simulink model "mcb_microchip_pmsm_foc_sensorless_SAME54"  (R2023b)
settings: Solver=FixedStepDiscrete  StartTime=0.0  StopTime=5  FixedStep=Ts  RelTol=1e-3  EnableMultiTasking=on
InitFcn:
  | mcb_microchip_pmsm_foc_sensorless_SAME54_data
values from neighbouring files (symbols this model uses):
  PI_params = mcb.internal.SetControllerParameters(pmsm,inverter,PU_System,T_pwm,2*Ts,Ts_speed)    [mcb_microchip_pmsm_foc_sensorless_SAME54_data.m]
  PU_System = mcb_SetPUSystem(pmsm,inverter)    [mcb_microchip_pmsm_foc_sensorless_SAME54_data.m]
  PWM_frequency = 12e3    (= 12000)    [mcb_microchip_pmsm_foc_sensorless_SAME54_data.m]
  Ts = T_pwm    (= 8.33333333333e-05)    [mcb_microchip_pmsm_foc_sensorless_SAME54_data.m]
  Ts_motor = T_pwm    (= 8.33333333333e-05)    [mcb_microchip_pmsm_foc_sensorless_SAME54_data.m]
  Ts_simulink = T_pwm    (= 8.33333333333e-05)    [mcb_microchip_pmsm_foc_sensorless_SAME54_data.m]
  Ts_speed = 10*Ts    (= 0.000833333333333)    [mcb_microchip_pmsm_foc_sensorless_SAME54_data.m]
  Vd_Ref_openLoop_PU = 0.15    [mcb_microchip_pmsm_foc_sensorless_SAME54_data.m]
undefined symbols (not defined in the file or in its folder): AIN0, AIN6, DiscIntNeverNeededParam, inverter, PA02, PA03, PA06, PA08, PA09, PA10, PA11, PA12, PA13, PA16, PA17, PA18, pad0, pad1, pad2, pad3, PB08, Pin, pmsm, SAME54P20A, Timer, TQFP128, VREFA, wo0, wo1, wo2, wo4, wo5, wo6
libraries: simulink x15, MCHP_Blockset x12, mcbcontrolslib x10, slpidlib x3, mcbpositiondecoderlib x2, mcbplantlib x1, autolibpmsmexterior x1
(part 3 of 4)

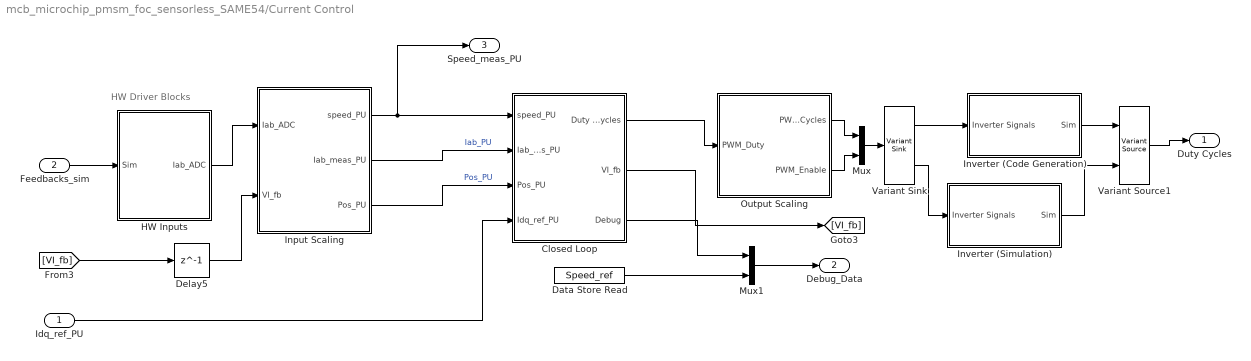
== system mcb_microchip_pmsm_foc_sensorless_SAME54/Current Control ==
  note: HW Driver Blocks
  Idq_ref_PU : Inport
  Feedbacks_sim : Inport  Port=2
  Closed Loop : Subsystem
  Data Store Read : DataStoreRead  DataStoreName=Speed_ref  DataStoreElements=Speed_ref  IndexOptions=Index vector (dialog)  Indices=1  OutputSizes=1
  Delay5 : Delay  DelayLength=1  SampleTime=Ts
  HW Inputs : Subsystem  Variant=on  VariantControlMode=sim codegen switching
  Input Scaling : Subsystem
  Inverter (Code Generation) : Subsystem
  Inverter (Simulation) : Subsystem
  Mux : Mux  Inputs=2
  Mux1 : Mux  Inputs=2
  Output Scaling : Subsystem
  Variant Sink : VariantSink  VariantControlMode=sim codegen switching
  Variant Source1 : VariantSource  VariantControlMode=sim codegen switching
  Duty Cycles : Outport  InitialOutput=0  VectorParamsAs1DForOutWhenUnconnected=off
  Debug_Data : Outport  Port=2
  Speed_meas_PU : Outport  Port=3  InitialOutput=0  VectorParamsAs1DForOutWhenUnconnected=off
  wires:
  Output Scaling/2(PWM_Enable) -> Mux/2
  Feedbacks_sim/1 -> HW Inputs/1(Sim)
  Input Scaling/2(Iab_meas_PU) -> Closed Loop/2(Iab_meas_PU)  "Iab_PU"
  Input Scaling/3(Pos_PU) -> Closed Loop/3(Pos_PU)  "Pos_PU"
  Variant Source1/1 -> Duty Cycles/1
  Output Scaling/1(PWM_Duty_Cycles) -> Mux/1
  Variant Sink/2 -> Inverter (Simulation)/1(Inverter Signals)
  Inverter (Code Generation)/1(Sim) -> Variant Source1/1
  Inverter (Simulation)/1(Sim) -> Variant Source1/2
  Variant Sink/1 -> Inverter (Code Generation)/1(Inverter Signals)
  Mux/1 -> Variant Sink/1
  HW Inputs/1(Iab_ADC) -> Input Scaling/1(Iab_ADC)
  [VI_fb] -> Delay5/1
  Delay5/1 -> Input Scaling/2(VI_fb)
  Mux1/1 -> Debug_Data/1
  Data Store Read/1 -> Mux1/2
  Input Scaling/1(speed_PU) -> Closed Loop/1(speed_PU), Speed_meas_PU/1
  Idq_ref_PU/1 -> Closed Loop/4(Idq_ref_PU)
  Closed Loop/1(Duty Cycles) -> Output Scaling/1(PWM_Duty)
  Closed Loop/2(VI_fb) -> [VI_fb]
  Closed Loop/3(Debug) -> Mux1/1

== system mcb_microchip_pmsm_foc_sensorless_SAME54/Heartbeat LED ==
  note: Heartbeat LED 1HZ
  Code generation : Subsystem
  RED_LED : Constant  OutDataTypeStr=uint16  SampleTime=0.1
  Simulation : Subsystem
  Variant Sink : VariantSink
  wires:
  RED_LED/1 -> Variant Sink/1
  Variant Sink/1 -> Code generation/1(In1)
  Variant Sink/2 -> Simulation/1(In1)

== system mcb_microchip_pmsm_foc_sensorless_SAME54/Inverter and Motor - Plant Model ==
  Duty_Cycles : Inport
  Plant Model : Subsystem  Variant=on  VariantControlMode=sim codegen switching  VariantControl=Variant1  PropagateVariantConditions=on
  Feedbacks_sim : Outport  VectorParamsAs1DForOutWhenUnconnected=off
  wires:
  Duty_Cycles/1 -> Plant Model/1(Duty_Cycles)
  Plant Model/1(Feedbacks_sim) -> Feedbacks_sim/1

== system mcb_microchip_pmsm_foc_sensorless_SAME54/Serial Receive ==
  CodeGen : Subsystem
  Data Store Write : DataStoreWrite  DataStoreName=Enable  IndexOptions=Index vector (dialog)  Indices=1  OutputSizes=1
  Sim : Subsystem
  Variant Source : VariantSource  VariantControlMode=sim codegen switching
  Variant Source1 : VariantSource  VariantControlMode=sim codegen switching
  SpeedRef : Outport
  wires:
  Variant Source/1 -> SpeedRef/1
  Variant Source1/1 -> Data Store Write/1
  Sim/1(SpeedRef) -> Variant Source/2
  Sim/2(Enable) -> Variant Source1/2
  CodeGen/1(SpeedRef) -> Variant Source/1
  CodeGen/2(Enable) -> Variant Source1/1

== system mcb_microchip_pmsm_foc_sensorless_SAME54/Speed Control ==
  SpeedRef : Inport
  Speed_Meas_PU : Inport  Port=2
  Data Store Write3 : DataStoreWrite  DataStoreName=Speed_ref  IndexOptions=Index vector (dialog)  Indices=1  OutputSizes=1
  Id_Ref : Constant  Value=0  OutDataTypeStr=dataType
  Mux : Mux  Inputs=2
  PI_Controller_Speed : Subsystem
  Speed_Ref_Selector : Subsystem
  IdqRef_PU : Outport  VectorParamsAs1DForOutWhenUnconnected=off
  wires:
  PI_Controller_Speed/1(Iq_ref) -> Mux/2
  Speed_Meas_PU/1 -> PI_Controller_Speed/2(N_fb)  "Speed_fb"
  Id_Ref/1 -> Mux/1
  Mux/1 -> IdqRef_PU/1
  Speed_Ref_Selector/1(Speed_Ref1) -> PI_Controller_Speed/1(N_ref)  "Speed_ref"
  SpeedRef/1 -> Data Store Write3/1, Speed_Ref_Selector/1(Speed_Ref)

== system mcb_microchip_pmsm_foc_sensorless_SAME54/Subsystem2 ==
  note: Fast Serial Data Monitoring (32-bit)
  Data_Log : Inport
  Counter Limited : simulink/Sources/Counter Limited  uplimit=59  tsamp=Ts_SerialCom
  Data : Subsystem  TreatAsAtomicUnit=on
  End : Subsystem  TreatAsAtomicUnit=on
  If : If  IfExpression=u1 == 0  ElseIfExpressions=u1 == 59
  Start : Subsystem  TreatAsAtomicUnit=on
  wires:
  Data_Log/1 -> Data/1(Data), Start/1(Data), End/1(Data)
  If/1 -> Start/Action
  If/2 -> End/Action
  Counter Limited/1 -> If/1
  If/3 -> Data/Action

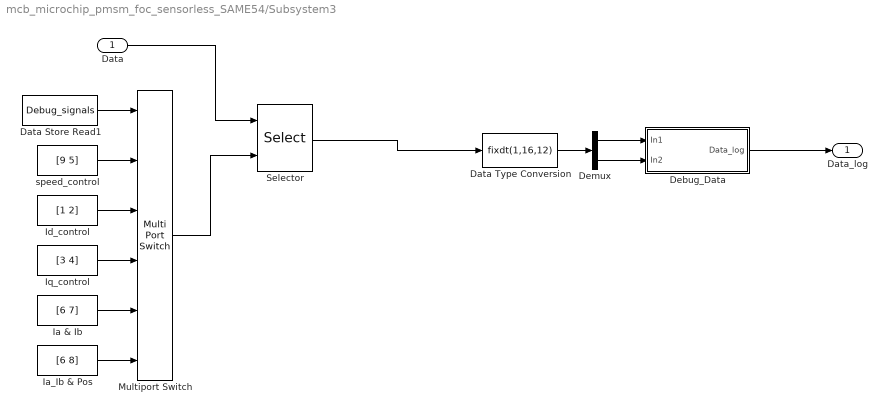
== system mcb_microchip_pmsm_foc_sensorless_SAME54/Subsystem3 ==
  Data : Inport
  Data Store Read1 : DataStoreRead  DataStoreName=Debug_signals  IndexOptions=Index vector (dialog)  Indices=1  OutputSizes=1
  Data Type Conversion : DataTypeConversion  OutDataTypeStr=fixdt(1,16,12)  RndMeth=Simplest  SaturateOnIntegerOverflow=off
  Debug_Data : Subsystem
  Demux : Demux  Outputs=2
  Ia & Ib : Constant  Value=[6 7]  OutDataTypeStr=uint16  SampleTime=-1
  Ia_Ib & Pos : Constant  Value=[6 8]  OutDataTypeStr=uint16  SampleTime=-1
  Id_control : Constant  Value=[1 2]  OutDataTypeStr=uint16  SampleTime=-1
  Iq_control : Constant  Value=[3 4]  OutDataTypeStr=uint16  SampleTime=-1
  Multiport Switch : MultiPortSwitch  Inputs=5  DiagnosticForDefault=Warning  OutDataTypeStr=uint16  RndMeth=Simplest  SaturateOnIntegerOverflow=off  InputSameDT=off
  Selector : Selector  InputPortWidth=9  IndexOptions=Index vector (port)  Indices=[1 3]  OutputSizes=1
  speed_control : Constant  Value=[9 5]  OutDataTypeStr=uint16  SampleTime=-1
  Data_log : Outport
  wires:
  Data Type Conversion/1 -> Demux/1
  Demux/2 -> Debug_Data/2(In2)
  Id_control/1 -> Multiport Switch/3
  Demux/1 -> Debug_Data/1(In1)
  Multiport Switch/1 -> Selector/2
  Ia & Ib/1 -> Multiport Switch/5
  Iq_control/1 -> Multiport Switch/4
  Ia_Ib & Pos/1 -> Multiport Switch/6
  Data/1 -> Selector/1
  speed_control/1 -> Multiport Switch/2
  Data Store Read1/1 -> Multiport Switch/1
  Selector/1 -> Data Type Conversion/1
  Debug_Data/1(Data_log) -> Data_log/1

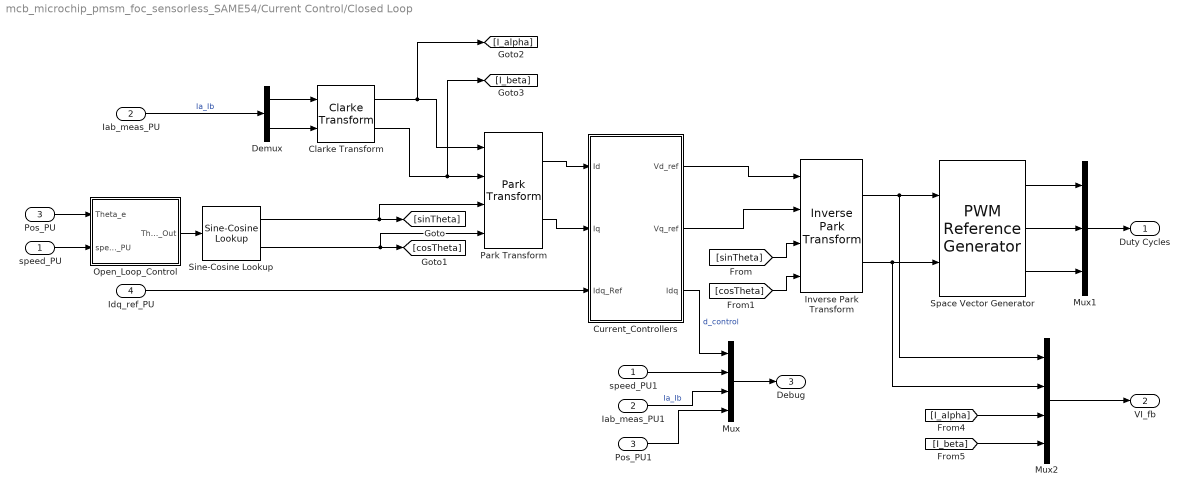
== system mcb_microchip_pmsm_foc_sensorless_SAME54/Current Control/Closed Loop ==
  speed_PU : Inport
  Iab_meas_PU : Inport  Port=2
  Pos_PU : Inport  Port=3
  Idq_ref_PU : Inport  Port=4
  Clarke Transform : mcbcontrolslib/Clarke Transform  VariantControl=Variant2  PhaseInput=Two inputs  EnPowerInv=off
  Current_Controllers : Subsystem
  Demux : Demux  Outputs=2
  Iab_meas_PU1 : InportShadow  Port=2
  Inverse Park Transform : mcbcontrolslib/Inverse Park Transform  PhaseInput=Two inputs  AxisAlignment=D-axis  ThetaInput=Sine and Cosine electrical position  AngleInput=Per-unit  N_points=1024
  Mux : Mux
  Mux1 : Mux  Inputs=3
  Mux2 : Mux
  Open_Loop_Control : Subsystem
  Park Transform : mcbcontrolslib/Park Transform  PhaseInput=Two inputs  AxisAlignment=D-axis  ThetaInput=Sine and Cosine electrical position  AngleInput=Per-unit  N_points=1024
  Pos_PU1 : InportShadow  Port=3
  Sine-Cosine Lookup : mcbcontrolslib/Sine-Cosine Lookup  AngleInput=Per-unit  N_points=1024
  Space Vector Generator : mcbcontrolslib/PWM Reference Generator  inSignal=Valphabeta  modType=SVM: space vector modulation
  speed_PU1 : InportShadow
  Duty Cycles : Outport  VectorParamsAs1DForOutWhenUnconnected=off
  VI_fb : Outport  Port=2  VectorParamsAs1DForOutWhenUnconnected=off
  Debug : Outport  Port=3  VectorParamsAs1DForOutWhenUnconnected=off
  wires:
  Current_Controllers/1(Vd_ref) -> Inverse Park Transform/1
  [cosTheta] -> Inverse Park Transform/4
  [I_beta] -> Mux2/4
  Inverse Park Transform/2 -> Space Vector Generator/2, Mux2/2
  Inverse Park Transform/1 -> Space Vector Generator/1, Mux2/1
  [sinTheta] -> Inverse Park Transform/3
  Mux2/1 -> VI_fb/1
  Clarke Transform/1 -> [I_alpha], Park Transform/1
  Current_Controllers/2(Vq_ref) -> Inverse Park Transform/2
  Clarke Transform/2 -> [I_beta], Park Transform/2
  [I_alpha] -> Mux2/3
  Space Vector Generator/1 -> Mux1/1
  Space Vector Generator/3 -> Mux1/3
  Mux1/1 -> Duty Cycles/1
  Space Vector Generator/2 -> Mux1/2
  Park Transform/1 -> Current_Controllers/1(Id)
  Park Transform/2 -> Current_Controllers/2(Iq)
  Demux/1 -> Clarke Transform/1
  Demux/2 -> Clarke Transform/2
  Iab_meas_PU/1 -> Demux/1  "Ia_Ib"
  Idq_ref_PU/1 -> Current_Controllers/3(Idq_Ref)
  Pos_PU/1 -> Open_Loop_Control/1(Theta_e)
  Open_Loop_Control/1(Theta_Out) -> Sine-Cosine Lookup/1
  speed_PU/1 -> Open_Loop_Control/2(speed_PU)
  speed_PU1/1 -> Mux/2
  Current_Controllers/3(Idq) -> Mux/1  "d_control"
  Mux/1 -> Debug/1
  Iab_meas_PU1/1 -> Mux/3  "Ia_Ib"
  Pos_PU1/1 -> Mux/4
  Sine-Cosine Lookup/2 -> Park Transform/4, [cosTheta]
  Sine-Cosine Lookup/1 -> Park Transform/3, [sinTheta]

== system mcb_microchip_pmsm_foc_sensorless_SAME54/Current Control/HW Inputs ==
  Sim : Inport
  Sensor Driver Blocks (codegen) : Subsystem  VariantControl=(codegen)
  Sensor Driver Blocks (sim) : Subsystem  VariantControl=(sim)
  Iab_ADC : Outport

== system mcb_microchip_pmsm_foc_sensorless_SAME54/Current Control/Input Scaling ==
  note: Current Measurements
  Iab_ADC : Inport
  VI_fb : Inport  Port=2
  Calculate Phase Currents : Subsystem
  Calculate position and speed : Subsystem
  speed_PU : Outport
  Iab_meas_PU : Outport  Port=2
  Pos_PU : Outport  Port=3
  wires:
  Calculate Phase Currents/1(Iab_meas_PU) -> Iab_meas_PU/1  "Iab_fb_PU"
  Iab_ADC/1 -> Calculate Phase Currents/1(Iab_ADC)
  VI_fb/1 -> Calculate position and speed/1(VI_fb)
  Calculate position and speed/2(speed_PU) -> speed_PU/1
  Calculate position and speed/1(Pos_PU) -> Pos_PU/1

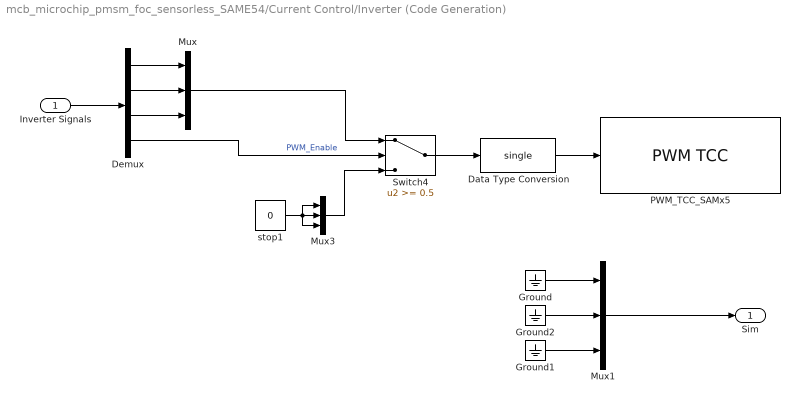
== system mcb_microchip_pmsm_foc_sensorless_SAME54/Current Control/Inverter (Code Generation) ==
  Inverter Signals : Inport
  Data Type Conversion : DataTypeConversion  OutDataTypeStr=single  SaturateOnIntegerOverflow=off  RndMeth=Floor
  Demux : Demux
  Ground : Ground
  Ground1 : Ground
  Ground2 : Ground
  Mux : Mux  Inputs=3
  Mux1 : Mux  Inputs=3
  Mux3 : Mux  Inputs=3
  PWM_TCC_SAMx5 : MCHP_Blockset/PWM IO/PWM TCC  TCCREF=TCC 0  WAVE_choice=Center aligned PWM  MaxPeriod_s=Ts  OTMX=Default  WO0=Dynamic Options  WO0_TXT=PA08 / Pin[33] / wo0  WO1=Dynamic Options  WO1_TXT=PA09 / Pin[34] / wo1  WO2=Dynamic Options  WO2_TXT=PA10 / Pin[35] / wo2  WO3=Dynamic Options  WO3_TXT=Not Used  WO4=Dynamic Options  WO4_TXT=PA16 / Pin[66] / wo4  WO5=Dynamic Options  WO5_TXT=PA17 / Pin[67] / wo5  WO6=Dynamic Options  WO6_TXT=PA18 / Pin[68] / wo6  WO7=Dynamic Options  WO7_TXT=Not Used  info=0  evalin_ws=PWM0max=MCHP_Fun.Hex2num('40B3870000000000');PWM0max=MCHP_Fun.Hex2num('40B3870000000000');PWM0max=MCHP_Fun.Hex2num('40B3870000000000');  SampleTime=Ts  MCHP_PORT={PWM0_H0}{TCC0_WO0}5:1:P8;{PWM0_H1}{TCC0_WO1}5:1:P9;{PWM0_H2}{TCC0_WO2}5:1:P10;{PWM0_L0}{TCC0_WO4}5:1:P16;{PWM0_L1}{TCC0_WO5}5:1:P17;{PWM0_L2}{TCC0_WO6}5:1:P18;  MCHP_MASTERLINK=mcb_microchip_pmsm_foc_sensorless_SAME54/Configurations/Microchip Master  INVEN_WO0=off  INVEN_WO1=off  INVEN_WO2=off  INVEN_WO3=off  INVEN_WO4=off  INVEN_WO5=off  INVEN_WO6=off  INVEN_WO7=off  SWAP_PWM0=off  SWAP_PWM1=off  SWAP_PWM2=off  SWAP_PWM3=off  POL_PWM0=off  POL_PWM1=off  POL_PWM2=off  POL_PWM3=off  POL_PWM4=off  POL_PWM5=off  InitPeriod_s=Ts  InitDutyCycle_s=0  InitDeadTimeH_s=1e-6  InitDeadTimeL_s=1e-6  InitOutputOverride=0  InitOutputOverride_val=0  BlockInput_VectorScalar=Vectors (grouped by function)  BlockInput_Period=Not a block input  BlockInput_DutyCycle=a Floating Point input within range [-1 1]  BlockInput_DeadTime=Not a block input  BlockInput_OutputOverride=Not a block input
      settings: SourceProductName=MPLAB Device Blocks for Simulink
  Switch4 : Switch  Threshold=0.5  RndMeth=Simplest  SaturateOnIntegerOverflow=off  InputSameDT=off
  stop1 : Constant  Value=0  OutDataTypeStr=dataType
  Sim : Outport  VectorParamsAs1DForOutWhenUnconnected=off
  wires:
  Inverter Signals/1 -> Demux/1
  Ground/1 -> Mux1/1
  Ground1/1 -> Mux1/3
  Ground2/1 -> Mux1/2
  Mux1/1 -> Sim/1
  Demux/1 -> Mux/1
  Demux/2 -> Mux/2
  Demux/3 -> Mux/3
  Switch4/1 -> Data Type Conversion/1
  Data Type Conversion/1 -> PWM_TCC_SAMx5/1
  stop1/1 -> Mux3/3, Mux3/2, Mux3/1
  Mux3/1 -> Switch4/3
  Demux/4 -> Switch4/2  "PWM_Enable"
  Mux/1 -> Switch4/1

== system mcb_microchip_pmsm_foc_sensorless_SAME54/Current Control/Inverter (Simulation) ==
  Inverter Signals : Inport
  Data Type Duplicate : DataTypeDuplicate
  Demux : Demux
  Mux : Mux  Inputs=3
  Mux2 : Mux  Inputs=3
  Subsystem : Subsystem
  Switch1 : Switch  Threshold=0.5  RndMeth=Simplest  SaturateOnIntegerOverflow=off  InputSameDT=off
  stop : Constant  Value=0  OutDataTypeStr=Inherit: Inherit via back propagation
  Sim : Outport  VectorParamsAs1DForOutWhenUnconnected=off
  wires:
  stop/1 -> Data Type Duplicate/2, Mux2/1, Mux2/3, Mux2/2
  Mux2/1 -> Switch1/3
  Switch1/1 -> Sim/1
  Inverter Signals/1 -> Demux/1
  Demux/4 -> Switch1/2  "PWM Enable"
  Mux/1 -> Subsystem/1(In1), Data Type Duplicate/1  "PWM Duty Cycles"
  Demux/1 -> Mux/1
  Demux/2 -> Mux/2
  Demux/3 -> Mux/3
  Subsystem/1(PWM_Duty_Cycles) -> Switch1/1  "test"

== system mcb_microchip_pmsm_foc_sensorless_SAME54/Current Control/Output Scaling ==
  PWM_Duty : Inport
  Constant2 : Constant  Value=0  OutDataTypeStr=Inherit: Inherit via back propagation
  Data Type Conversion : DataTypeConversion  OutDataTypeStr=dataType  SaturateOnIntegerOverflow=off  RndMeth=Floor
  Enable : DataStoreRead  DataStoreName=Enable  IndexOptions=Index vector (dialog)  Indices=1  OutputSizes=1
  Mode Selector : Subsystem
  Mux1 : Mux  Inputs=3
  Switch for Current offset calibration : Switch  Criteria=u2 ~= 0  Threshold=250  SaturateOnIntegerOverflow=off  InputSameDT=off
  PWM_Duty_Cycles : Outport
  PWM_Enable : Outport  Port=2
  wires:
  Data Type Conversion/1 -> PWM_Enable/1
  Enable/1 -> Data Type Conversion/1
  PWM_Duty/1 -> Switch for Current offset calibration/3
  Mode Selector/1(CurrentOffsetEn) -> Switch for Current offset calibration/2
  Mux1/1 -> Switch for Current offset calibration/1
  Constant2/1 -> Mux1/3, Mux1/2, Mux1/1
  Switch for Current offset calibration/1 -> PWM_Duty_Cycles/1

== system mcb_microchip_pmsm_foc_sensorless_SAME54/Heartbeat LED/Code generation ==
  In1 : Inport
  DBG LED 1 : MCHP_Blockset/Digital IO/Digital Output Write  PORT=Dynamic Options  PORT_TXT="B   [ 0 : 31 ]"  PIN=27  PACK=off  SIMULTANEOUS=off  ORDERING=None  SampleTime=-1  MCHP_PORT={Digital Out}{DOU}1:1:B27;  MCHP_MASTERLINK=mcb_microchip_pmsm_foc_sensorless_SAME54/Configurations/Microchip Master
      settings: SourceProductName=MPLAB Device Blocks for Simulink
  Delay 10Hz : Delay  DelayLength=1  InitialCondition=0  SampleTime=0.25
  Logical Operator : Logic  Operator=NOT  AllPortsSameDT=off  OutDataTypeStr=boolean
  Terminator : Terminator
  wires:
  Logical Operator/1 -> DBG LED 1/1, Delay 10Hz/1
  Delay 10Hz/1 -> Logical Operator/1
  In1/1 -> Terminator/1

== system mcb_microchip_pmsm_foc_sensorless_SAME54/Heartbeat LED/Simulation ==
  In1 : Inport
  Simulation_Terminator : Terminator
  wires:
  In1/1 -> Simulation_Terminator/1

== system mcb_microchip_pmsm_foc_sensorless_SAME54/Inverter and Motor - Plant Model/Plant Model ==
  Duty_Cycles : Inport
  Inverter and Motor (codegen) : Subsystem  VariantControl=(codegen)
  Inverter and Motor (sim) : Subsystem  VariantControl=(sim)
  Feedbacks_sim : Outport  VectorParamsAs1DForOutWhenUnconnected=off

== system mcb_microchip_pmsm_foc_sensorless_SAME54/Serial Receive/CodeGen ==
  Data Store Write1 : DataStoreWrite  DataStoreName=Debug_signals  IndexOptions=Index vector (dialog)  Indices=1  OutputSizes=1
  Data Type Conversion : DataTypeConversion  OutDataTypeStr=uint16  SaturateOnIntegerOverflow=off  RndMeth=Floor
  Subsystem : Subsystem
  Subsystem1 : Subsystem
  UART Rx : MCHP_Blockset/BUS UART/UART Rx  UART_REF=2  Flag_Out=on  Rx_Size_popup=User defined  Rx_Size=1  S_Rx_Size=1  Split=Read all received char  SplitChar=10  OutputDefault_popup=do nothing (end of output vector will be undefined)  OutputDefault=-2  ORDERING=None  SampleTime=.001  MCHP_MASTERLINK=mcb_microchip_pmsm_foc_sensorless_SAME54/Configurations/Microchip Master  MCHP_COMPILED_INFO="CompiledSampleTime= [0.0010000000000000000208   0 ];CompiledInportDataTypes=[    ];CompiledInportDataWidth=[];"
      settings: SourceProductName=MPLAB Device Blocks for Simulink
  SpeedRef : Outport
  Enable : Outport  Port=2
  wires:
  UART Rx/1 -> Data Type Conversion/1
  Subsystem/3(Debug Signal Selection) -> Data Store Write1/1
  UART Rx/2 -> Subsystem1/1(In1)
  Subsystem/2(Enable) -> Enable/1
  Subsystem/1(SpeedRef) -> SpeedRef/1
  Subsystem1/2(Data out) -> Subsystem/1(In1)
  Subsystem1/1(NewData) -> Subsystem/Enable
  Data Type Conversion/1 -> Subsystem1/Enable

== system mcb_microchip_pmsm_foc_sensorless_SAME54/Serial Receive/Sim ==
  Data Type Conversion1 : DataTypeConversion  OutDataTypeStr=dataType  RndMeth=Simplest  SaturateOnIntegerOverflow=off
  Data Type Conversion2 : DataTypeConversion  OutDataTypeStr=boolean  RndMeth=Simplest  SaturateOnIntegerOverflow=off
  Gain : Gain  Gain=1/PU_System.N_base  RndMeth=Simplest  OutDataTypeStr=Inherit: Same as input
  Speed Ref [RPM] : Step  Time=3.5  Before=0.2 * PU_System.N_base  After=0.8 * PU_System.N_base  OutDataTypeStr=single  SampleTime=0.001
  Step1 : Step  OutDataTypeStr=single  SampleTime=0.001
  SpeedRef : Outport
  Enable : Outport  Port=2
  wires:
  Speed Ref [RPM]/1 -> Gain/1
  Data Type Conversion1/1 -> SpeedRef/1
  Step1/1 -> Data Type Conversion2/1
  Data Type Conversion2/1 -> Enable/1
  Gain/1 -> Data Type Conversion1/1

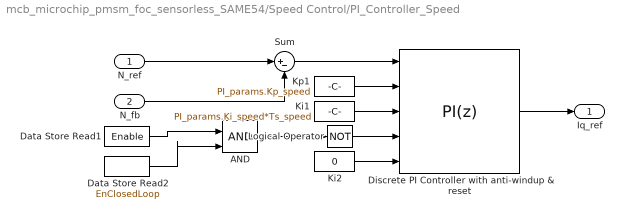
== system mcb_microchip_pmsm_foc_sensorless_SAME54/Speed Control/PI_Controller_Speed ==
  N_ref : Inport
  N_fb : Inport  Port=2
  AND : Logic  IconShape=distinctive  AllPortsSameDT=off  OutDataTypeStr=boolean
  Data Store Read2 : DataStoreRead  DataStoreName=EnClosedLoop  IndexOptions=Index vector (dialog)  Indices=1  OutputSizes=1
  Data Store Read1 : DataStoreRead  DataStoreName=Enable  IndexOptions=Index vector (dialog)  Indices=1  OutputSizes=1
  Discrete PI Controller with anti-windup & reset : slpidlib/PID Controller  Controller=PI  Form=Parallel  TimeDomain=Discrete-time  UseExternalTs=off  SampleTime=-1  IntegratorMethod=Forward Euler  FilterMethod=Forward Euler  ControllerParametersSource=external  P=1  I=1  UseKiTs=on  D=0  N=100  UseFilter=on  TunerSelectOption=Transfer Function Based (PID Tuner App)  InitialConditionSource=external  InitialConditionForIntegrator=0  InitialConditionForFilter=0  DifferentiatorICPrevScaledInput=0  ExternalReset=level  TrackingMode=off  Kt=1  LimitOutput=on  SatLimitsSource=internal  UpperSaturationLimit=1  LowerSaturationLimit=-1  LinearizeAsGain=on  AntiWindupMode=clamping  Kb=1  LimitIntegrator=off  UpperIntegratorSaturationLimit=inf  LowerIntegratorSaturationLimit=-inf  RndMeth=Simplest  POutMin=[]  POutMax=[]  IOutMin=[]  IOutMax=[]  DOutMin=[]  DOutMax=[]  NOutMin=[]  NOutMax=[]  SumOutMin=[]  SumOutMax=[]  SaturationOutDataTypeStr=Inherit: Inherit via back propagation  SaturationOutMin=[]  SaturationOutMax=[]  PParamMin=[]  PParamMax=[]  IParamMin=[]  IParamMax=[]  DParamMin=[]  DParamMax=[]  NParamMin=[]  NParamMax=[]  KbParamMin=[]  KbParamMax=[]  KtParamMin=[]  KtParamMax=[]  KbOutMin=[]  KbOutMax=[]  KtOutMin=[]  KtOutMax=[]  IntegratorOutMin=[]  IntegratorOutMax=[]  FilterOutMin=[]  FilterOutMax=[]  SumI1OutMin=[]  SumI1OutMax=[]  SumI2OutMin=[]  SumI2OutMax=[]  SumI3OutMin=[]  SumI3OutMax=[]  SumI4OutMin=[]  SumI4OutMax=[]  SumDOutMin=[]  SumDOutMax=[]  DifferentiatorOutMin=[]  DifferentiatorOutMax=[]  FilterDiffOutCoefMin=[]  FilterDiffOutCoefMax=[]  ReciprocalOutMin=[]  ReciprocalOutMax=[]  SumDenOutMin=[]  SumDenOutMax=[]  SumNumOutMin=[]  SumNumOutMax=[]  DivideOutMin=[]  DivideOutMax=[]  UdiffTsProdOutMin=[]  UdiffTsProdOutMax=[]  NTsProdOutMin=[]  NTsProdOutMax=[]  UintegralTsProdOutMin=[]  UintegralTsProdOutMax=[]  UngainTsProdOutMin=[]  UngainTsProdOutMax=[]  ClampingZeroOutDataTypeStr=Inherit: Inherit via back propagation  ClampingZeroOutMin=[]  ClampingZeroOutMax=[]  FilterDenConstantOutDataTypeStr=Inherit: Inherit via back propagation  FilterDenConstantOutMin=[]  FilterDenConstantOutMax=[]  PCopyOutDataTypeStr=Inherit: Inherit via back propagation  PCopyOutMin=[]  PCopyOutMax=[]  NCopyOutDataTypeStr=Inherit: Inherit via back propagation  NCopyOutMin=[]  NCopyOutMax=[]  IntegratorContinuousStateAttributes=''  IntegratorStateMustResolveToSignalObject=off  IntegratorRTWStateStorageClass=Auto  FilterContinuousStateAttributes=''  FilterStateMustResolveToSignalObject=off  FilterRTWStateStorageClass=Auto  ParallelPVariant=ExternalParameters  IdealPVariant=Disabled  IVariant=ExternalParameters  DVariant=Disabled  IntegratorVariant=Discrete  SatVariant=Enabled  AWVariant=DiscClampingParallel  PCopyVariant=Disabled  TRVariant=Disabled  FdbkBlocksVariant=Forward  IdealPFdbkVariant=Disabled  SatFdbkVariant=Disabled  DerivativeFilterVariant=Disabled  NVariant=Disabled  NCopyVariant=Disabled_SignalSpec  FilterICVariant=Disabled  IntegratorICVariant=ExternalICs  ExternalResetVariant=ExternalReset  TRSumVariant=Passthrough  SumFdbkVariant=Disabled  SumVariant=Sum_PI  TsampFilterVariant=InternalTs  TsampNgainVariant=Passthrough  TsampIntegralVariant=Disabled_SignalSpec  ExternalSaturationOutDataTypeStr=Inherit: Same as second input
      settings: LibrarySourceBlock=mcbcontrolslib/PI Controller
  Ki1 : Constant  Value=PI_params.Ki_speed*Ts_speed  OutDataTypeStr=dataType  SampleTime=-1
  Ki2 : Constant  Value=0  OutDataTypeStr=dataType  SampleTime=-1
  Kp1 : Constant  Value=PI_params.Kp_speed  OutDataTypeStr=dataType  SampleTime=-1
  Logical Operator : Logic  Operator=NOT  IconShape=distinctive  AllPortsSameDT=off  OutDataTypeStr=boolean
  Sum : Sum  Inputs=|+-  OutDataTypeStr=Inherit: Same as first input
  Iq_ref : Outport  VectorParamsAs1DForOutWhenUnconnected=off
  wires:
  Discrete PI Controller with anti-windup & reset/1 -> Iq_ref/1
  Ki1/1 -> Discrete PI Controller with anti-windup & reset/3
  Kp1/1 -> Discrete PI Controller with anti-windup & reset/2
  N_fb/1 -> Sum/2
  N_ref/1 -> Sum/1
  Sum/1 -> Discrete PI Controller with anti-windup & reset/1
  Logical Operator/1 -> Discrete PI Controller with anti-windup & reset/4
  Ki2/1 -> Discrete PI Controller with anti-windup & reset/5
  Data Store Read1/1 -> AND/1
  Data Store Read2/1 -> AND/2
  AND/1 -> Logical Operator/1

== system mcb_microchip_pmsm_foc_sensorless_SAME54/Speed Control/Speed_Ref_Selector ==
  Speed_Ref : Inport
  Constant : Constant  Value=0.1  OutDataTypeStr=dataType
  Constant1 : Constant  Value=-0.1  OutDataTypeStr=dataType
  Data Store Read : DataStoreRead  DataStoreName=Speed_ref  IndexOptions=Index vector (dialog)  Indices=1  OutputSizes=1
  Data Store Read1 : DataStoreRead  DataStoreName=EnClosedLoop  IndexOptions=Index vector (dialog)  Indices=1  OutputSizes=1
  IIR Filter : mcbcontrolslib/IIR Filter  VariantControl=Low Pass Filter  VariantSelect=Low-pass  Filter_constant=0.001*(Ts_speed/Ts)  advancedSettings=off  Ts=50e-6  cutOff_freq=38.6611
  Switch : Switch  Criteria=u2 > Threshold  SaturateOnIntegerOverflow=off  InputSameDT=off
  Switch1 : Switch  Criteria=u2 > Threshold  SaturateOnIntegerOverflow=off  InputSameDT=off
  Speed_Ref1 : Outport
  wires:
  IIR Filter/1 -> Speed_Ref1/1  "Speed_Ref"
  Data Store Read1/1 -> Switch/2
  Switch/1 -> IIR Filter/1  "Speed_Ref"
  Constant/1 -> Switch1/1
  Data Store Read/1 -> Switch1/2
  Switch1/1 -> Switch/3
  Speed_Ref/1 -> Switch/1
  Constant1/1 -> Switch1/3

== system mcb_microchip_pmsm_foc_sensorless_SAME54/Subsystem2/Data ==
  Data : Inport
  Action Port : ActionPort  ActionPortLabel=else
  UART Tx : MCHP_Blockset/BUS UART/UART Tx  UART_REF=2  ORDERING=None  AllOrNothing=off  SampleTime=-1  MCHP_MASTERLINK=mcb_microchip_pmsm_foc_sensorless_SAME54/Configurations/Microchip Master  NSend_Input=off  UART_String=off  NSend_Output=off
      settings: SourceProductName=MPLAB Device Blocks for Simulink
  wires:
  Data/1 -> UART Tx/1

== system mcb_microchip_pmsm_foc_sensorless_SAME54/Subsystem2/End ==
  Data : Inport
  Action Port : ActionPort  ActionPortLabel=elseif(u1 == 59)
  Mux : Mux  Inputs=2
  Start : Constant  Value=hex2dec('45')  OutDataTypeStr=uint8
  UART Tx : MCHP_Blockset/BUS UART/UART Tx  UART_REF=2  ORDERING=None  AllOrNothing=off  SampleTime=-1  MCHP_MASTERLINK=mcb_microchip_pmsm_foc_sensorless_SAME54/Configurations/Microchip Master  NSend_Input=off  UART_String=off  NSend_Output=off
      settings: SourceProductName=MPLAB Device Blocks for Simulink
  wires:
  Start/1 -> Mux/2
  Data/1 -> Mux/1
  Mux/1 -> UART Tx/1

== system mcb_microchip_pmsm_foc_sensorless_SAME54/Subsystem2/Start ==
  Data : Inport
  Action Port : ActionPort  ActionPortLabel=if(u1 == 0)
  End : Constant  Value=hex2dec('53')  OutDataTypeStr=uint8
  Mux : Mux  Inputs=2
  UART Tx : MCHP_Blockset/BUS UART/UART Tx  UART_REF=2  ORDERING=None  AllOrNothing=off  SampleTime=-1  MCHP_MASTERLINK=mcb_microchip_pmsm_foc_sensorless_SAME54/Configurations/Microchip Master  NSend_Input=off  UART_String=off  NSend_Output=off
      settings: SourceProductName=MPLAB Device Blocks for Simulink
  wires:
  End/1 -> Mux/1
  Data/1 -> Mux/2
  Mux/1 -> UART Tx/1

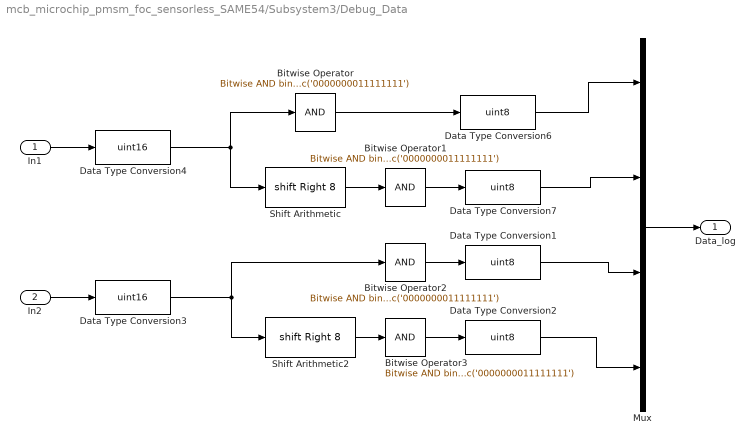
== system mcb_microchip_pmsm_foc_sensorless_SAME54/Subsystem3/Debug_Data ==
  In1 : Inport
  In2 : Inport  Port=2
  Bitwise Operator{,1..3} (4 alike) : simulink/Logic and Bit Operations/Bitwise Operator  logicop=AND  UseBitMask=on  BitMask=bin2dec('0000000011111111')  BitMaskRealWorld=Stored Integer
  Data Type Conversion{1..2,6..7} (4 alike) : DataTypeConversion  OutDataTypeStr=uint8  RndMeth=Simplest  SaturateOnIntegerOverflow=off
  Data Type Conversion3 : DataTypeConversion  OutDataTypeStr=uint16  ConvertRealWorld=Stored Integer (SI)  RndMeth=Simplest  SaturateOnIntegerOverflow=off
  Data Type Conversion4 : DataTypeConversion  OutDataTypeStr=uint16  ConvertRealWorld=Stored Integer (SI)  RndMeth=Simplest  SaturateOnIntegerOverflow=off
  Mux : Mux
  Shift Arithmetic : ArithShift  BitShiftNumber=8  BitShiftDirection=Right
  Shift Arithmetic2 : ArithShift  BitShiftNumber=8  BitShiftDirection=Right
  Data_log : Outport
  wires:
  Mux/1 -> Data_log/1
  In1/1 -> Data Type Conversion4/1
  Data Type Conversion4/1 -> Shift Arithmetic/1, Bitwise Operator/1
  Data Type Conversion6/1 -> Mux/1
  Data Type Conversion7/1 -> Mux/2
  Bitwise Operator2/1 -> Data Type Conversion1/1
  Data Type Conversion1/1 -> Mux/3
  Bitwise Operator/1 -> Data Type Conversion6/1
  Shift Arithmetic/1 -> Bitwise Operator1/1
  Data Type Conversion2/1 -> Mux/4
  Bitwise Operator1/1 -> Data Type Conversion7/1
  Shift Arithmetic2/1 -> Bitwise Operator3/1
  Bitwise Operator3/1 -> Data Type Conversion2/1
  Data Type Conversion3/1 -> Shift Arithmetic2/1, Bitwise Operator2/1
  In2/1 -> Data Type Conversion3/1

== system mcb_microchip_pmsm_foc_sensorless_SAME54/Current Control/Closed Loop/Current_Controllers ==
  Id : Inport
  Iq : Inport  Port=2
  Idq_Ref : Inport  Port=3
  DQ Limiter : mcbcontrolslib/DQ Limiter  satMethodInputType=Specify via dialog  satMethodSelected=D-Q equivalence  satLimitInputType=Specify via dialog  Vmax=1
  Demux : Demux  Outputs=2
  Mux : Mux
  PI_Controller_Id : Subsystem
  PI_Controller_Iq : Subsystem
  Terminator : Terminator
  Vd_ref : Outport  VectorParamsAs1DForOutWhenUnconnected=off
  Vq_ref : Outport  Port=2  VectorParamsAs1DForOutWhenUnconnected=off
  Idq : Outport  Port=3  VectorParamsAs1DForOutWhenUnconnected=off
  wires:
  Iq/1 -> Mux/4, PI_Controller_Iq/2(I_fb)  "Iq_fb"
  PI_Controller_Id/1(V_ref) -> DQ Limiter/1
  Id/1 -> PI_Controller_Id/2(I_fb), Mux/2  "Id_fb"
  Demux/1 -> PI_Controller_Id/1(I_ref), Mux/1  "Id_Ref"
  Demux/2 -> Mux/3, PI_Controller_Iq/1(I_ref)  "Iq_Ref"
  DQ Limiter/1 -> Vd_ref/1
  DQ Limiter/2 -> Vq_ref/1
  PI_Controller_Iq/1(V_ref) -> DQ Limiter/2
  DQ Limiter/3 -> Terminator/1
  Idq_Ref/1 -> Demux/1
  Mux/1 -> Idq/1

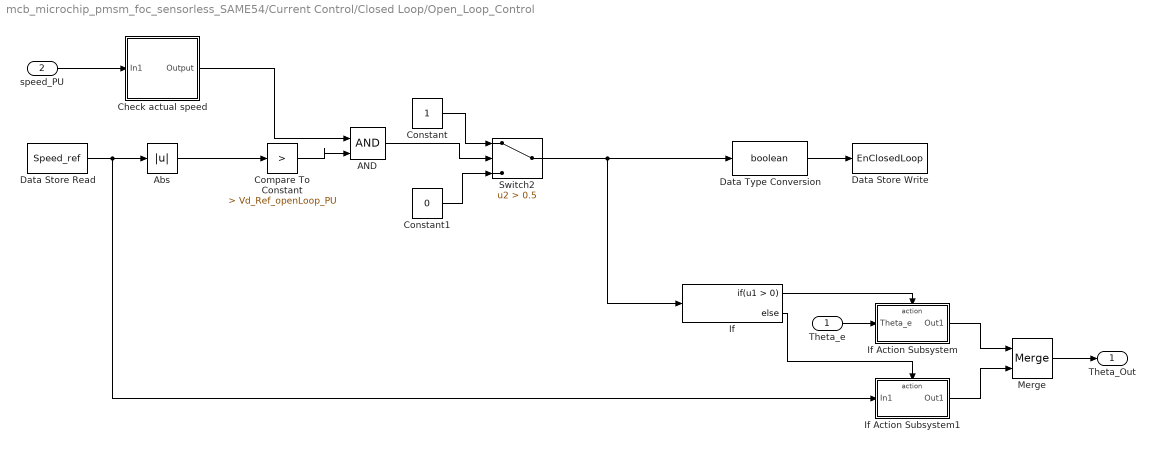
== system mcb_microchip_pmsm_foc_sensorless_SAME54/Current Control/Closed Loop/Open_Loop_Control ==
  Theta_e : Inport
  speed_PU : Inport  Port=2
  AND : Logic  IconShape=distinctive  AllPortsSameDT=off  OutDataTypeStr=boolean
  Abs : Abs  SaturateOnIntegerOverflow=off
  Check actual speed : Subsystem
  Compare To Constant : simulink/Logic and Bit Operations/Compare To Constant  relop=>  const=Vd_Ref_openLoop_PU  OutDataTypeStr=boolean
  Constant : Constant  OutDataTypeStr=uint16
  Constant1 : Constant  Value=0  OutDataTypeStr=uint16
  Data Store Read : DataStoreRead  DataStoreName=Speed_ref  IndexOptions=Index vector (dialog)  Indices=1  OutputSizes=1
  Data Store Write : DataStoreWrite  DataStoreName=EnClosedLoop  IndexOptions=Index vector (dialog)  Indices=1  OutputSizes=1
  Data Type Conversion : DataTypeConversion  OutDataTypeStr=boolean  RndMeth=Simplest  SaturateOnIntegerOverflow=off
  If : If
  If Action Subsystem : Subsystem  TreatAsAtomicUnit=on
  If Action Subsystem1 : Subsystem  TreatAsAtomicUnit=on
  Merge : Merge
  Switch2 : Switch  Criteria=u2 > Threshold  Threshold=0.5  SaturateOnIntegerOverflow=off  InputSameDT=off
  Theta_Out : Outport
  wires:
  Constant1/1 -> Switch2/3
  Constant/1 -> Switch2/1
  Abs/1 -> Compare To Constant/1
  Data Store Read/1 -> If Action Subsystem1/1(In1), Abs/1
  Data Type Conversion/1 -> Data Store Write/1
  Compare To Constant/1 -> AND/2
  AND/1 -> Switch2/2
  speed_PU/1 -> Check actual speed/1(In1)
  Check actual speed/1(Output) -> AND/1
  If/1 -> If Action Subsystem/Action
  If/2 -> If Action Subsystem1/Action
  Theta_e/1 -> If Action Subsystem/1(Theta_e)
  If Action Subsystem/1(Out1) -> Merge/1
  If Action Subsystem1/1(Out1) -> Merge/2
  Merge/1 -> Theta_Out/1
  Switch2/1 -> If/1, Data Type Conversion/1

== system mcb_microchip_pmsm_foc_sensorless_SAME54/Current Control/HW Inputs/Sensor Driver Blocks (codegen) ==
  Sim : Inport
  ADC SAMx5 : MCHP_Blockset/Analog IO/ADC SAMx5 SAMC2x  ADCREF=ADC 0 and ADC 1 (slave)  VREF_seq0=Dynamic Options  VREF_seq0_TXT=PA03 / VREFA / Pin[10]  info=0  SampleTime=Ts  MCHP_PORT={ADC0_seq0.0}{ADC0_AIN0}15:2:P2;{ADC0_seq0.1}{ADC0_AIN6}15:2:P6;{ADC1_seq0.0}{ADC1_AIN0}15:2:P40;  MCHP_MASTERLINK=mcb_microchip_pmsm_foc_sensorless_SAME54/Configurations/Microchip Master  MCHP_CRC=4740560  TrigSource_seq0=Dynamic Options  TrigSource_seq0_TXT=TCC0 PWM event Overflow - Period  ADC0_seq0=Dynamic Options  ADC0_seq0_TXT=PA02 / AIN0 / Pin[9]  ADC1_seq0=Dynamic Options  ADC1_seq0_TXT=PB08 / AIN0 / Pin[19]  ADC0_seq0_1=Dynamic Options  ADC0_seq0_1_TXT=PA06 / AIN6 / Pin[23]  ADC1_seq0_1=Dynamic Options  ADC1_seq0_1_TXT=Not Used  ADC0_seq0_2=Dynamic Options  ADC0_seq0_2_TXT=Not Used  ADC1_seq0_2=Dynamic Options  ADC1_seq0_2_TXT=Not Used  ADC0_seq0_3=Dynamic Options  ADC0_seq0_3_TXT=Not Used  ADC1_seq0_3=Dynamic Options  ADC1_seq0_3_TXT=Not Used  ADC0_seq0_4=Dynamic Options  ADC0_seq0_4_TXT=Not Used  ADC1_seq0_4=Dynamic Options  ADC1_seq0_4_TXT=Not Used  ADC0_seq0_5=Dynamic Options  ADC0_seq0_5_TXT=Not Used  ADC1_seq0_5=Dynamic Options  ADC1_seq0_5_TXT=Not Used  Resolution_seq0=12 bits  SampleTime_seq0_s=1e-6  TrigTimeStep_seq0=on  info_seq0=0  TrigSource_seq1=Dynamic Options  TrigSource_seq1_TXT=after this block evaluation  ADC0_seq1=Dynamic Options  ADC0_seq1_TXT=Not Used  ADC1_seq1=Dynamic Options  ADC1_seq1_TXT=Not Used  ADC0_seq1_1=Dynamic Options  ADC0_seq1_1_TXT=Not Used  ADC1_seq1_1=Dynamic Options  ADC1_seq1_1_TXT=Not Used  ADC0_seq1_2=Dynamic Options  ADC0_seq1_2_TXT=Not Used  ADC1_seq1_2=Dynamic Options  ADC1_seq1_2_TXT=Not Used  ADC0_seq1_3=Dynamic Options  ADC0_seq1_3_TXT=Not Used  ADC1_seq1_3=Dynamic Options  ADC1_seq1_3_TXT=Not Used  ADC0_seq1_4=Dynamic Options  ADC0_seq1_4_TXT=Not Used  ADC1_seq1_4=Dynamic Options  ADC1_seq1_4_TXT=Not Used  ADC0_seq1_5=Dynamic Options  ADC0_seq1_5_TXT=Not Used  ADC1_seq1_5=Dynamic Options  ADC1_seq1_5_TXT=Not Used  Resolution_seq1=12 bits  SampleTime_seq1_s=1e-6  TrigTimeStep_seq1=on  info_seq1=0  TrigSource_seq2=Dynamic Options  TrigSource_seq2_TXT=after this block evaluation  ADC0_seq2=Dynamic Options  ADC0_seq2_TXT=Not Used  ADC1_seq2=Dynamic Options  ADC1_seq2_TXT=Not Used  ADC0_seq2_1=Dynamic Options  ADC0_seq2_1_TXT=Not Used  ADC1_seq2_1=Dynamic Options  ADC1_seq2_1_TXT=Not Used  ADC0_seq2_2=Dynamic Options  ADC0_seq2_2_TXT=Not Used  ADC1_seq2_2=Dynamic Options  ADC1_seq2_2_TXT=Not Used  ADC0_seq2_3=Dynamic Options  ADC0_seq2_3_TXT=Not Used  ADC1_seq2_3=Dynamic Options  ADC1_seq2_3_TXT=Not Used  ADC0_seq2_4=Dynamic Options  ADC0_seq2_4_TXT=Not Used  ADC1_seq2_4=Dynamic Options  ADC1_seq2_4_TXT=Not Used  ADC0_seq2_5=Dynamic Options  ADC0_seq2_5_TXT=Not Used  ADC1_seq2_5=Dynamic Options  ADC1_seq2_5_TXT=Not Used  Resolution_seq2=12 bits  SampleTime_seq2_s=1e-6  TrigTimeStep_seq2=off  info_seq2=0  TrigSource_seq3=Dynamic Options  TrigSource_seq3_TXT=after this block evaluation  ADC0_seq3=Dynamic Options  ADC0_seq3_TXT=Not Used  ADC1_seq3=Dynamic Options  ADC1_seq3_TXT=Not Used  ADC0_seq3_1=Dynamic Options  ADC0_seq3_1_TXT=Not Used  ADC1_seq3_1=Dynamic Options  ADC1_seq3_1_TXT=Not Used  ADC0_seq3_2=Dynamic Options  ADC0_seq3_2_TXT=Not Used  ADC1_seq3_2=Dynamic Options  ADC1_seq3_2_TXT=Not Used  ADC0_seq3_3=Dynamic Options  ADC0_seq3_3_TXT=Not Used  ADC1_seq3_3=Dynamic Options  ADC1_seq3_3_TXT=Not Used  ADC0_seq3_4=Dynamic Options  ADC0_seq3_4_TXT=Not Used  ADC1_seq3_4=Dynamic Options  ADC1_seq3_4_TXT=Not Used  ADC0_seq3_5=Dynamic Options  ADC0_seq3_5_TXT=Not Used  ADC1_seq3_5=Dynamic Options  ADC1_seq3_5_TXT=Not Used  Resolution_seq3=12 bits  SampleTime_seq3_s=1e-6  TrigTimeStep_seq3=off  info_seq3=0  TrigSource_seq4=Dynamic Options  TrigSource_seq4_TXT=after this block evaluation  ADC0_seq4=Dynamic Options  ADC0_seq4_TXT=Not Used  ADC1_seq4=Dynamic Options  ADC1_seq4_TXT=Not Used  ADC0_seq4_1=Dynamic Options  ADC0_seq4_1_TXT=Not Used  ADC1_seq4_1=Dynamic Options  ADC1_seq4_1_TXT=Not Used  ADC0_seq4_2=Dynamic Options  ADC0_seq4_2_TXT=Not Used  ADC1_seq4_2=Dynamic Options  ADC1_seq4_2_TXT=Not Used  ADC0_seq4_3=Dynamic Options  ADC0_seq4_3_TXT=Not Used  ADC1_seq4_3=Dynamic Options  ADC1_seq4_3_TXT=Not Used  ADC0_seq4_4=Dynamic Options  ADC0_seq4_4_TXT=Not Used  ADC1_seq4_4=Dynamic Options  ADC1_seq4_4_TXT=Not Used  ADC0_seq4_5=Dynamic Options  ADC0_seq4_5_TXT=Not Used  ADC1_seq4_5=Dynamic Options  ADC1_seq4_5_TXT=Not Used  Resolution_seq4=12 bits  SampleTime_seq4_s=1e-6  TrigTimeStep_seq4=off  info_seq4=0  TrigSource_seq5=Dynamic Options  TrigSource_seq5_TXT=after this block evaluation  ADC0_seq5=Dynamic Options  ADC0_seq5_TXT=Not Used  ADC1_seq5=Dynamic Options  ADC1_seq5_TXT=Not Used  ADC0_seq5_1=Dynamic Options  ADC0_seq5_1_TXT=Not Used  ADC1_seq5_1=Dynamic Options  ADC1_seq5_1_TXT=Not Used  ADC0_seq5_2=Dynamic Options  ADC0_seq5_2_TXT=Not Used  ADC1_seq5_2=Dynamic Options  ADC1_seq5_2_TXT=Not Used  ADC0_seq5_3=Dynamic Options  ADC0_seq5_3_TXT=Not Used  ADC1_seq5_3=Dynamic Options  ADC1_seq5_3_TXT=Not Used  ADC0_seq5_4=Dynamic Options  ADC0_seq5_4_TXT=Not Used  ADC1_seq5_4=Dynamic Options  ADC1_seq5_4_TXT=Not Used  ADC0_seq5_5=Dynamic Options  ADC0_seq5_5_TXT=Not Used  ADC1_seq5_5=Dynamic Options  ADC1_seq5_5_TXT=Not Used  Resolution_seq5=12 bits  SampleTime_seq5_s=1e-6  TrigTimeStep_seq5=off  info_seq5=0
      settings: SourceProductName=MPLAB Device Blocks for Simulink
  Data Store Write : DataStoreWrite  Commented=on  DataStoreName=Speed_ref  IndexOptions=Index vector (dialog)  Indices=1  OutputSizes=1
  Data Type Conversion : DataTypeConversion  OutDataTypeStr=single  RndMeth=Simplest  SaturateOnIntegerOverflow=off
  Gain1 : Gain  Gain=1/4095  OutDataTypeStr=Inherit: Same as input  ParamDataTypeStr=Inherit: Same as input
  Mux : Mux  Inputs=2
  Terminator : Terminator
  Terminator1 : Terminator
  Iab_ADC : Outport
  wires:
  Sim/1 -> Terminator/1
  Mux/1 -> Iab_ADC/1
  ADC SAMx5/1 -> Mux/1
  ADC SAMx5/2 -> Mux/2
  Gain1/1 -> Terminator1/1
  Data Type Conversion/1 -> Gain1/1
  ADC SAMx5/3 -> Data Type Conversion/1

== system mcb_microchip_pmsm_foc_sensorless_SAME54/Current Control/HW Inputs/Sensor Driver Blocks (sim) ==
  Sim : Inport
  Iab_ADC : Outport
  wires:
  Sim/1 -> Iab_ADC/1

== system mcb_microchip_pmsm_foc_sensorless_SAME54/Current Control/Input Scaling/Calculate Phase Currents ==
  Iab_ADC : Inport
  Add : Sum  Inputs=+-
  Data Store Read2 : DataStoreRead  DataStoreName=EnCurOffset  IndexOptions=Index vector (dialog)  Indices=1  OutputSizes=1
  Data Type Conversion : DataTypeConversion  OutDataTypeStr=int32  ConvertRealWorld=Stored Integer (SI)  SaturateOnIntegerOverflow=off  RndMeth=Floor
  Data Type Conversion1 : DataTypeConversion  OutDataTypeStr=dataType  SaturateOnIntegerOverflow=off  RndMeth=Floor
  Data Type Conversion2 : DataTypeConversion  Commented=on  OutDataTypeStr=uint16  SaturateOnIntegerOverflow=off  RndMeth=Floor
  Demux1 : Demux  Commented=on  Outputs=2
  Demux2 : Demux  Commented=on  Outputs=2
  Gain1 : Gain  Gain=1/2048  OutDataTypeStr=Inherit: Same as input  ParamDataTypeStr=Inherit: Same as input
  Offset : Subsystem
  UART Tx-Matlab4 : MCHP_Blockset/BUS UART/UART Tx-Matlab  Commented=on  UART_REF=2  CHANNELS=[1 2]  AllOrNothing=on  SampleTime=-1  MCHP_MASTERLINK=mcb_microchip_pmsm_foc_sensorless_SAME54/Configurations/Microchip Master  MCHP_COMPILED_INFO="CompiledSampleTime= [8.3333333333333330551e-05   0 ];CompiledInportDataTypes=[  5   5 ];CompiledInportDataWidth=[1  1];"
      settings: SourceProductName=MPLAB Device Blocks for Simulink
  Iab_meas_PU : Outport  VectorParamsAs1DForOutWhenUnconnected=off
  wires:
  Add/1 -> Data Type Conversion1/1
  Iab_ADC/1 -> Demux2/1, Data Type Conversion/1  "U2 CH2"
  Data Type Conversion1/1 -> Gain1/1
  Data Store Read2/1 -> Offset/Enable
  Data Type Conversion/1 -> Add/1, Offset/1(Iab)
  Offset/1(Offset) -> Add/2
  Gain1/1 -> Data Type Conversion2/1, Iab_meas_PU/1
  Demux1/1 -> UART Tx-Matlab4/1  "U2 CH1"
  Demux2/1 -> UART Tx-Matlab4/2  "U2 CH2"
  Data Type Conversion2/1 -> Demux1/1

== system mcb_microchip_pmsm_foc_sensorless_SAME54/Current Control/Input Scaling/Calculate position and speed ==
  VI_fb : Inport
  Demux : Demux  Outputs=2
  Sliding Mode Observer : Subsystem
  Pos_PU : Outport
  speed_PU : Outport  Port=2
  wires:
  VI_fb/1 -> Sliding Mode Observer/1(InputSignals)
  Demux/1 -> Pos_PU/1
  Demux/2 -> speed_PU/1
  Sliding Mode Observer/1(Position/Speed) -> Demux/1

== system mcb_microchip_pmsm_foc_sensorless_SAME54/Current Control/Inverter (Simulation)/Subsystem ==
  In1 : Inport
  Constant : Constant  Value=0.5  OutDataTypeStr=dataType
  Gain : Gain  Gain=0.5  OutDataTypeStr=Inherit: Same as input
  Sum : Sum  Inputs=|++
  PWM_Duty_Cycles : Outport
  wires:
  Gain/1 -> Sum/1
  Constant/1 -> Sum/2
  In1/1 -> Gain/1
  Sum/1 -> PWM_Duty_Cycles/1  "PWM_Duty_Cycles"

== system mcb_microchip_pmsm_foc_sensorless_SAME54/Current Control/Output Scaling/Mode Selector ==
  Delay : Delay  DelayLength=1
  NOT : Logic  Operator=NOT  IconShape=distinctive  AllPortsSameDT=off  OutDataTypeStr=boolean
  Subsystem1 : Subsystem
  Up Counter : Subsystem
  CurrentOffsetEn : Outport
  wires:
  Up Counter/1(Count) -> Subsystem1/1(Count)
  Delay/1 -> NOT/1
  NOT/1 -> Up Counter/Enable
  Subsystem1/2(EnClosedLoop) -> Delay/1
  Subsystem1/1(Current Offset) -> CurrentOffsetEn/1

== system mcb_microchip_pmsm_foc_sensorless_SAME54/Inverter and Motor - Plant Model/Plant Model/Inverter and Motor (codegen) ==
  Duty_Cycles : Inport
  Ground : Ground
  Terminator : Terminator
  Feedbacks_sim : Outport  VectorParamsAs1DForOutWhenUnconnected=off
  wires:
  Duty_Cycles/1 -> Terminator/1
  Ground/1 -> Feedbacks_sim/1

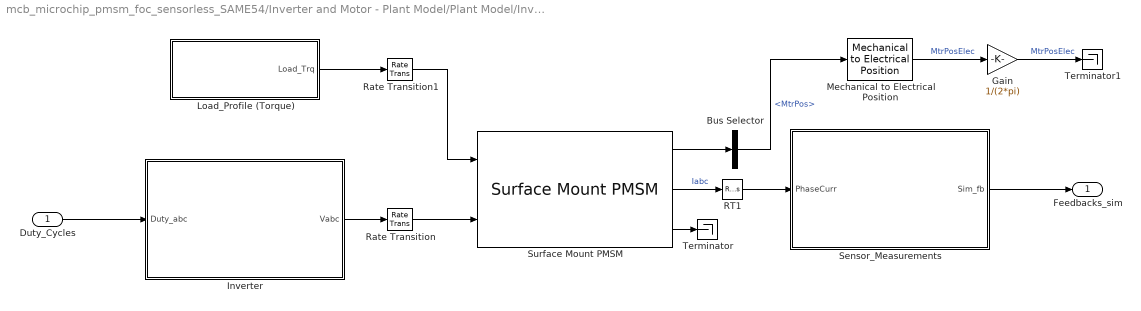
== system mcb_microchip_pmsm_foc_sensorless_SAME54/Inverter and Motor - Plant Model/Plant Model/Inverter and Motor (sim) ==
  Duty_Cycles : Inport
  Bus Selector : BusSelector  OutputSignals=MtrPos
  Gain : Gain  Gain=1/(2*pi)  OutDataTypeStr=Inherit: Same as input
  Inverter : Subsystem
  Load_Profile (Torque) : Subsystem
  Mechanical to Electrical Position : mcbpositiondecoderlib/Mechanical to Electrical Position  PolePairsInputType=Specify via dialog  NrPP=pmsm.p  selectedRange=Radians  MechOfstInputType=Specify via dialog  mechOffsetIn=0  maxAngleIn=2*pi  InputDataType=single  VariantSelect=floating-point
  RT1 : RateTransition  Deterministic=off  OutPortSampleTime=Ts_simulink
  Rate Transition : RateTransition  Deterministic=off  OutPortSampleTime=Ts_motor
  Rate Transition1 : RateTransition  Deterministic=off  OutPortSampleTime=Ts_motor
  Sensor_Measurements : Subsystem
  Surface Mount PMSM : autolibpmsmexterior/Surface Mount PMSM  port_config=Torque  sim_type=Discrete  Ts=Ts_motor  FilePath=surfacepmsm_motordata.m  P=pmsm.p  Rs=pmsm.Rs + inverter.R_board  Ldq_=pmsm.Ld  KConstText=Permanent flux linkage constant (lambda_pm):  lambda_pm=pmsm.FluxPM  Ke=159.9771  Kt=1.323  mechanical=[pmsm.J, pmsm.B, 0]  idq0=[0 0]  theta_init=0  omega_init=0  KConst=pmsm.FluxPM  lambda_pm_calc=pmsm.FluxPM  RefBlkName='autolibpmsmexterior/Surface Mount PMSM'  aMode=5  Ldq="[0.00078136  0.00078136]"
  Terminator : Terminator
  Terminator1 : Terminator
  Feedbacks_sim : Outport  VectorParamsAs1DForOutWhenUnconnected=off
  wires:
  Inverter/1(Vabc) -> Rate Transition/1
  Surface Mount PMSM/2 -> RT1/1  "Iabc"
  Sensor_Measurements/1(Sim_fb) -> Feedbacks_sim/1
  Surface Mount PMSM/3 -> Terminator/1
  Load_Profile (Torque)/1(Load_Trq) -> Rate Transition1/1
  Duty_Cycles/1 -> Inverter/1(Duty_abc)
  Rate Transition/1 -> Surface Mount PMSM/2
  Rate Transition1/1 -> Surface Mount PMSM/1
  RT1/1 -> Sensor_Measurements/1(PhaseCurr)
  Gain/1 -> Terminator1/1  "MtrPosElec"
  Mechanical to Electrical Position/1 -> Gain/1  "MtrPosElec"
  Bus Selector/1 -> Mechanical to Electrical Position/1  "<MtrPos>"
  Surface Mount PMSM/1 -> Bus Selector/1

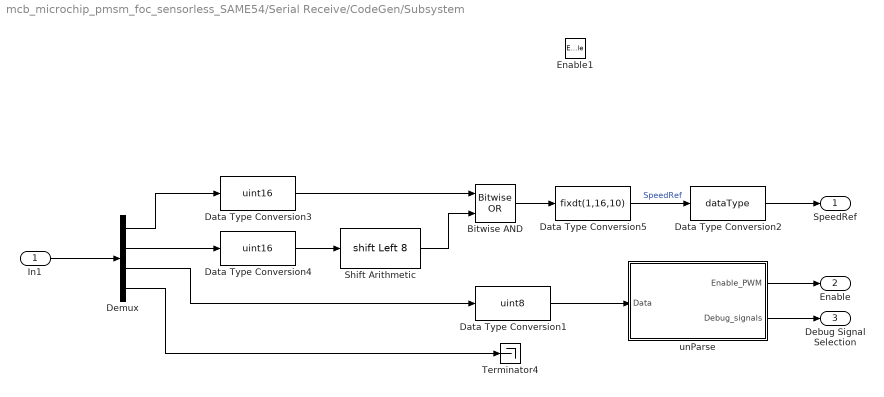
== system mcb_microchip_pmsm_foc_sensorless_SAME54/Serial Receive/CodeGen/Subsystem ==
  In1 : Inport
  Enable1 : EnablePort
  Bitwise AND : simulink/Logic and Bit Operations/Bitwise Operator  logicop=OR  UseBitMask=off  NumInputPorts=2  BitMask=bin2dec('11011001')  BitMaskRealWorld=Stored Integer
  Data Type Conversion1 : DataTypeConversion  OutDataTypeStr=uint8  RndMeth=Simplest  SaturateOnIntegerOverflow=off
  Data Type Conversion2 : DataTypeConversion  OutDataTypeStr=dataType  RndMeth=Simplest  SaturateOnIntegerOverflow=off
  Data Type Conversion3 : DataTypeConversion  OutDataTypeStr=uint16  RndMeth=Simplest  SaturateOnIntegerOverflow=off
  Data Type Conversion4 : DataTypeConversion  OutDataTypeStr=uint16  RndMeth=Simplest  SaturateOnIntegerOverflow=off
  Data Type Conversion5 : DataTypeConversion  OutDataTypeStr=fixdt(1,16,10)  ConvertRealWorld=Stored Integer (SI)  SaturateOnIntegerOverflow=off
  Demux : Demux
  Shift Arithmetic : ArithShift  BitShiftNumber=8  BitShiftDirection=Left
  Terminator4 : Terminator
  unParse : Subsystem
  SpeedRef : Outport
  Enable : Outport  Port=2
  Debug Signal Selection : Outport  Port=3
  wires:
  Data Type Conversion4/1 -> Shift Arithmetic/1
  Data Type Conversion3/1 -> Bitwise AND/1
  In1/1 -> Demux/1
  unParse/2(Debug_signals) -> Debug Signal Selection/1
  Data Type Conversion2/1 -> SpeedRef/1
  Demux/3 -> Data Type Conversion1/1
  Bitwise AND/1 -> Data Type Conversion5/1
  unParse/1(Enable_PWM) -> Enable/1
  Data Type Conversion1/1 -> unParse/1(Data)
  Demux/2 -> Data Type Conversion4/1
  Demux/4 -> Terminator4/1
  Shift Arithmetic/1 -> Bitwise AND/2
  Data Type Conversion5/1 -> Data Type Conversion2/1  "SpeedRef"
  Demux/1 -> Data Type Conversion3/1

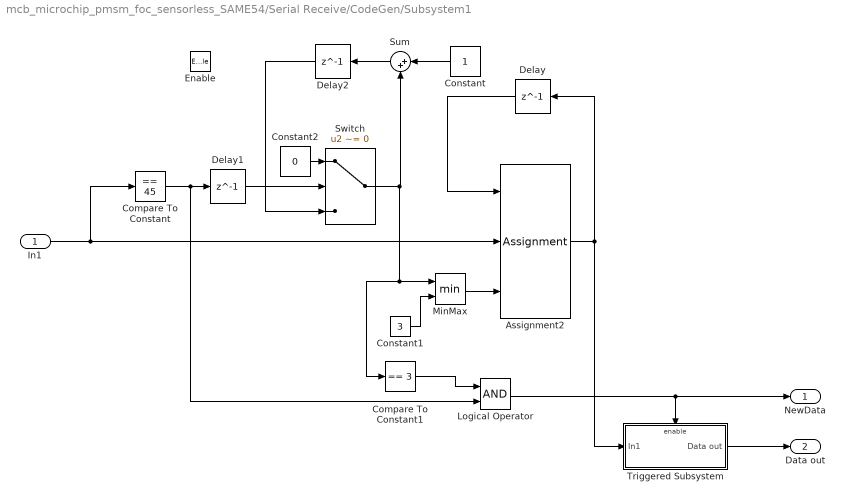
== system mcb_microchip_pmsm_foc_sensorless_SAME54/Serial Receive/CodeGen/Subsystem1 ==
  In1 : Inport
  Enable : EnablePort
  Assignment2 : Assignment  IndexMode=Zero-based  DiagnosticForDimensions=Warning  IndexOptions=Starting index (port)  Indices=1  OutputSizes=1
  Compare To Constant : simulink/Logic and Bit Operations/Compare To Constant  relop===  const=45  OutDataTypeStr=boolean
  Compare To Constant1 : simulink/Logic and Bit Operations/Compare To Constant  relop===  const=3  OutDataTypeStr=boolean
  Constant : Constant  OutDataTypeStr=uint16  SampleTime=-1
  Constant1 : Constant  Value=3  OutDataTypeStr=uint16  SampleTime=-1
  Constant2 : Constant  Value=0  OutDataTypeStr=uint16  SampleTime=-1
  Delay : Delay  DelayLength=1  InitialCondition=[0 0 0 0]
  Delay1 : Delay  DelayLength=1  InitialCondition=0
  Delay2 : Delay  DelayLength=1  InitialCondition=0
  Logical Operator : Logic  AllPortsSameDT=off  OutDataTypeStr=boolean
  MinMax : MinMax  Inputs=2
  Sum : Sum  Inputs=|++
  Switch : Switch  Criteria=u2 ~= 0  SaturateOnIntegerOverflow=off  InputSameDT=off
  Triggered Subsystem : Subsystem  TreatAsAtomicUnit=on
  NewData : Outport  OutputWhenDisabled=reset  InitialOutput=0
  Data out : Outport  Port=2
  wires:
  Logical Operator/1 -> Triggered Subsystem/Enable, NewData/1
  Triggered Subsystem/1(Data out) -> Data out/1
  Constant2/1 -> Switch/1
  Delay1/1 -> Switch/2
  Switch/1 -> MinMax/1, Compare To Constant1/1, Sum/2
  Sum/1 -> Delay2/1
  MinMax/1 -> Assignment2/3
  Constant1/1 -> MinMax/2
  Constant/1 -> Sum/1
  In1/1 -> Assignment2/2, Compare To Constant/1
  Compare To Constant1/1 -> Logical Operator/1
  Compare To Constant/1 -> Delay1/1, Logical Operator/2
  Delay2/1 -> Switch/3
  Delay/1 -> Assignment2/1
  Assignment2/1 -> Delay/1, Triggered Subsystem/1(In1)
